simulink model "Energy_Cost"  (Simulink 8.8)
settings: Solver=ode23t  StartTime=0.0  StopTime=24  RelTol=1e-3  EnableMultiTasking=on
model workspace: external: MAT-File (data not in the file)
libraries: simulink x4
(part 1 of 5)
settings Model: Creator=jm3gonza  LastModifiedBy=Lenio
settings DataIOCC: LimitDataPoints=off  SaveOutput=off
settings OptimizationCC: ExpressionDepthLimit=2147483647
settings DebuggingCC: AlgebraicLoopMsg=none  UnconnectedInputMsg=none  UnconnectedOutputMsg=none  UnconnectedLineMsg=none

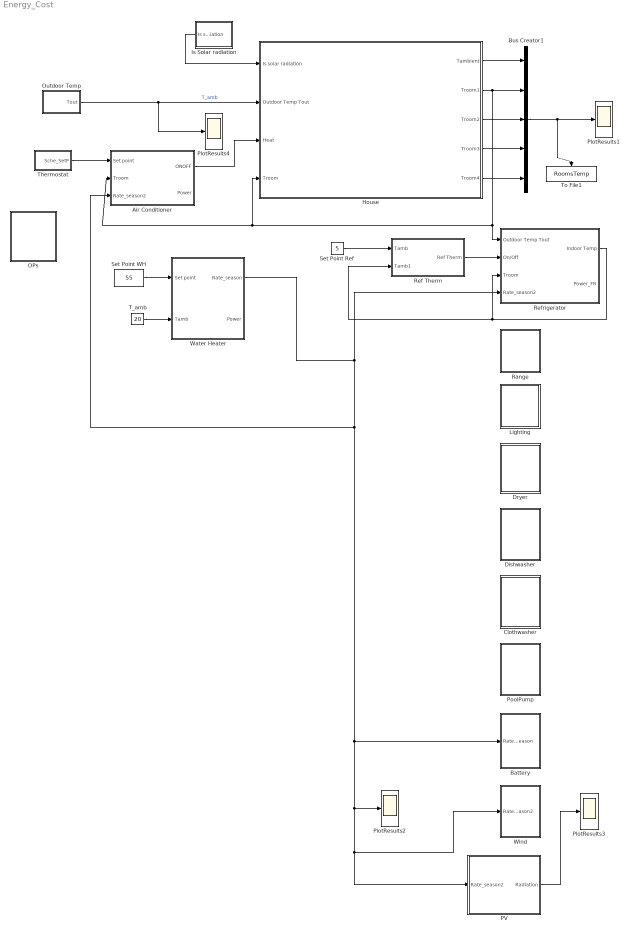
== system Energy_Cost ==
  Air Conditioner : Subsystem
  Battery : Subsystem
  Bus Creator1 : BusCreator  Inputs=5
  Clothwasher : Subsystem
  Dishwasher : Subsystem
  Dryer : Subsystem
  House : Subsystem
  Is Solar radiation : Subsystem
  Lighting : Subsystem
  OPs : Subsystem
  Outdoor Temp : Subsystem
  PV : Subsystem
  PlotResults{1..4} (4 alike) : Scope
  PoolPump : Subsystem
  Range : Subsystem
  Ref Therm : Subsystem
  Refrigerator : Subsystem
  Set Point Ref : Constant  Value=5
  Set Point WH : Constant  Value=55
  T_amb : Constant  Value=20
  Thermostat : Subsystem
  To File1 : ToFile  Filename=RoomsTemp  MatrixName=RoomsTemp
  Water Heater : Subsystem
  Wind : Subsystem
  wires:
  Set Point WH/1 -> Water Heater/1(Set point)
  T_amb/1 -> Water Heater/2(Tamb)
  Outdoor Temp/1(Tout) -> PlotResults4/1, House/2(Outdoor Temp Tout)  "T_amb"
  House/5(Troom4) -> Bus Creator1/5
  House/1(Tambient) -> Bus Creator1/1
  House/2(Troom1) -> Bus Creator1/2, Refrigerator/1(Outdoor Temp Tout), House/4(Troom), Air Conditioner/2(Troom)
  House/3(Troom2) -> Bus Creator1/3
  House/4(Troom3) -> Bus Creator1/4
  Bus Creator1/1 -> To File1/1, PlotResults1/1
  Air Conditioner/1(ONOFF) -> House/3(Heat)
  Is Solar radiation/1(Is solar radiation) -> House/1(Is solar radiation)
  Thermostat/1(Sche_SetP) -> Air Conditioner/1(Set point)
  Set Point Ref/1 -> Ref Therm/1(Tamb)
  Ref Therm/1(Ref Therm) -> Refrigerator/2(On/Off)
  Refrigerator/1(Indoor Temp) -> Refrigerator/3(Troom), Ref Therm/2(Tamb1)
  Water Heater/1(Rate_season) -> Refrigerator/4(Rate_season2), Air Conditioner/3(Rate_season2), Wind/1(Rate_season2), PV/1(Rate_season2), PlotResults2/1, Battery/1(Rate_season)
  PV/1(Radiation) -> PlotResults3/1

== system Energy_Cost/Air Conditioner ==
  Set point : Inport
  Troom : Inport  Port=2
  Rate_season2 : Inport  Port=3
  AA or Heat : Constant
  AA_OnOff : Constant
  Cost_AA : Subsystem
  PlotResults4 : Scope
  Q_AC : Constant  Value=-50644783.1184
  Relay : Relay  OnSwitchValue=0.5  OffSwitchValue=-0.5
  Sum : Sum  Inputs=|+-  SampleTime=0  SaturateOnIntegerOverflow=on  InputSameDT=on  OutDataTypeStr=Inherit: Same as first input
  a : Product  Inputs=3  RndMeth=Zero
  ONOFF : Outport  InitialOutput=0
  Power : Outport  Port=2  InitialOutput=0
  wires:
  Set point/1 -> Sum/1
  Troom/1 -> Sum/2
  Sum/1 -> Relay/1
  Relay/1 -> a/1, PlotResults4/1
  a/1 -> ONOFF/1, Cost_AA/1(Powe_cons)
  Q_AC/1 -> a/2
  AA_OnOff/1 -> a/3
  Rate_season2/1 -> Cost_AA/2(Rate_season2)
  Cost_AA/1(Power) -> Power/1

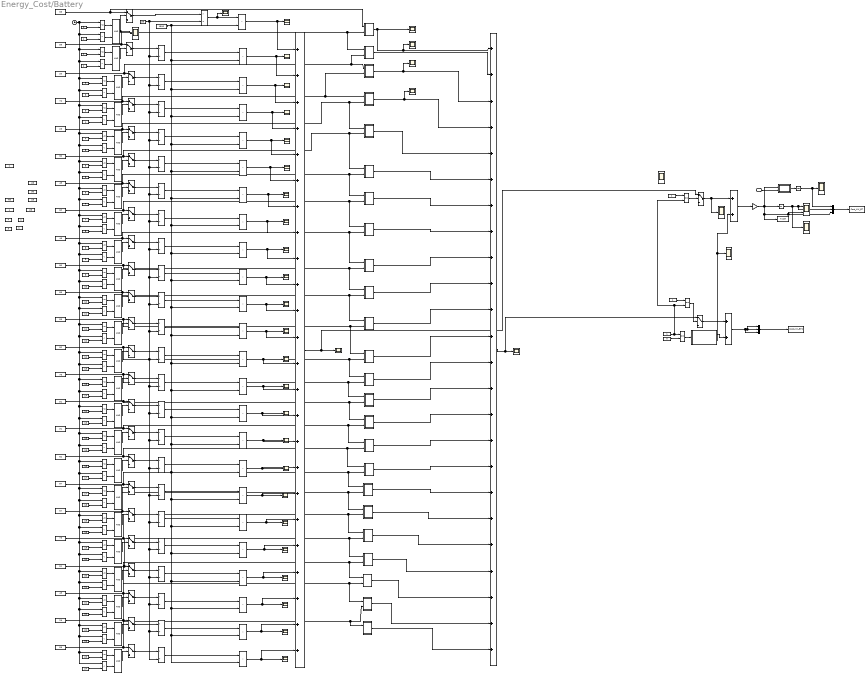
== system Energy_Cost/Battery ==
  Rate_season : Inport
  Add1 : Sum  Inputs=++++++++++++++++++++++++
  Add2 : Sum  Inputs=++++++++++++++++++++++++
  Add8 : Sum
  Add9 : Sum
  BT_OnOff : Constant
  Battery_type : Constant
  Bus Creator1 : BusCreator  Inputs=3
  Bus Creator4 : BusCreator  Inputs=3
  Clock1 : Clock
  Default : Constant  Value=0
  Divide{2..25} (24 alike) : Product  Inputs=*/
  Dot Product{1,3..25} (24 alike) : DotProduct  InputSameDT=on  OutDataTypeStr=Inherit: Inherit via internal rule
  Enabled Subsystem1 : Subsystem  TreatAsAtomicUnit=on
  Gain : Gain  Gain=.001
  Integrator : Integrator
  Integrator3 : Integrator
  Load Value : Constant  Value=-60
  LoadsDay : Constant
  Logical Operator{1..18,20..25} (24 alike) : Logic  AllPortsSameDT=off  OutDataTypeStr=boolean
  MinOfLoad : Constant  Value=30
  PlotResults{1..4,6,8} (6 alike) : Scope
  PlotResults5 : Scope  NumInputPorts=2
  Power1 : Constant  Value=35
  Power10 : Constant  Value=80
  Power11 : Constant  Value=85
  Power12 : Constant  Value=55
  Power13 : Constant  Value=92
  Power14 : Constant  Value=76
  Power15 : Constant  Value=51
  Power16 : Constant  Value=31
  Power17 : Constant  Value=62
  Power18 : Constant  Value=87
  Power19 : Constant  Value=97
  Power2 : Constant  Value=55
  Power20 : Constant  Value=75
  Power21 : Constant  Value=61
  Power22 : Constant  Value=43
  Power23 : Constant  Value=29
  Power24 : Constant  Value=59
  Power25 : Constant  Value=1500
  Power3 : Constant  Value=20
  Power4 : Constant  Value=70
  Power5 : Constant  Value=25
  Power6 : Constant  Value=30
  Power7 : Constant  Value=45
  Power8 : Constant  Value=60
  Power9 : Constant  Value=45
  Rates : Subsystem
  Relational Operator1 : RelationalOperator  Operator===  RndMeth=Nearest  InputSameDT=on
  Relational Operator{6..7,10..11,14..15,18..19,22..23,27..28,31..32,35..36,39..40,43..44,47..48,51..52} (24 alike) : RelationalOperator  RndMeth=Nearest  InputSameDT=on
  Relational Operator103 : RelationalOperator  Operator===  RndMeth=Nearest  InputSameDT=on
  Relational Operator{8..9,12..13,16..17,20..21,25..26,29..30,33..34,37..38,41..42,45..46,49..50,53..54} (24 alike) : RelationalOperator  Operator=<  RndMeth=Nearest  InputSameDT=on
  Relational Operator55 : RelationalOperator  Operator===  RndMeth=Nearest  InputSameDT=on
  Subsystem : Subsystem
  Subsystem1 : Subsystem
  Subsystem10 : Subsystem
  Subsystem11 : Subsystem
  Subsystem12 : Subsystem
  Subsystem13 : Subsystem
  Subsystem14 : Subsystem
  Subsystem15 : Subsystem
  Subsystem16 : Subsystem
  Subsystem17 : Subsystem
  Subsystem18 : Subsystem
  Subsystem19 : Subsystem
  Subsystem2 : Subsystem
  Subsystem20 : Subsystem
  Subsystem21 : Subsystem
  Subsystem22 : Subsystem
  Subsystem23 : Subsystem
  Subsystem3 : Subsystem
  Subsystem4 : Subsystem
  Subsystem5 : Subsystem
  Subsystem6 : Subsystem
  Subsystem7 : Subsystem
  Subsystem8 : Subsystem
  Subsystem9 : Subsystem
  Switch{1,7..29,31..32} (26 alike) : Switch  Criteria=u2 > Threshold
  To File1 : ToFile  Filename=TinBT  MatrixName=TinBT
  To File3 : ToFile  Filename=Cost_KW_BT2  MatrixName=Cost_KW_BT2
  To File5 : ToFile  Filename=Cost_KW_BT  MatrixName=Cost_KW_BT
  Type1 : Constant
  Type10 : Constant  Value=2
  Type11 : Constant  Value=3
  Type12 : Constant  Value=4
  Type13 : Constant  Value=4
  Type14 : Constant  Value=5
  Type15 : Constant  Value=6
  Type16 : Constant  Value=5
  Type17 : Constant  Value=6
  Type18 : Constant  Value=7
  Type19 : Constant  Value=8
  Type2 : Constant  Value=2
  Type20 : Constant  Value=8
  Type21 : Constant  Value=9
  Type22 : Constant  Value=10
  Type23 : Constant  Value=9
  Type24 : Constant  Value=7
  Type25 : Constant  Value=10
  Type26 : Constant  Value=11
  Type27 : Constant  Value=12
  Type28 : Constant  Value=12
  Type29 : Constant  Value=13
  Type3 : Constant  Value=3
  Type30 : Constant  Value=14
  Type31 : Constant  Value=13
  Type32 : Constant  Value=14
  Type33 : Constant  Value=15
  Type34 : Constant  Value=16
  Type35 : Constant  Value=16
  Type36 : Constant  Value=17
  Type37 : Constant  Value=18
  Type38 : Constant  Value=17
  Type39 : Constant  Value=15
  Type4 : Constant  Value=4
  Type40 : Constant  Value=11
  Type41 : Constant  Value=18
  Type42 : Constant  Value=19
  Type43 : Constant  Value=20
  Type44 : Constant  Value=20
  Type45 : Constant  Value=21
  Type46 : Constant  Value=22
  Type47 : Constant  Value=21
  Type48 : Constant  Value=22
  Type49 : Constant  Value=23
  Type5 : Constant
  Type50 : Constant  Value=24
  Type52 : Constant  Value=35
  Type55 : Constant  Value=23
  Type56 : Constant  Value=19
  Type6 : Constant  Value=0
  Type7 : Constant
  Type8 : Constant  Value=2
  Type9 : Constant  Value=3
  WhenUsed1 : Constant  Value=25
  WhenUsed2 : Constant  Value=25
  WhenUsed3 : Constant  Value=25
  radiation : Constant
  radiation1 : Constant
  scope{1..26} (26 alike) : Scope
  soc{,1..4} (5 alike) : Scope
  wires:
  Integrator/1 -> Bus Creator4/1, PlotResults3/1
  Rates/1(Rate) -> Integrator/1
  Integrator3/1 -> PlotResults6/1, Bus Creator4/2, PlotResults5/1  "kw-hr"
  Bus Creator4/1 -> To File5/1
  Rate_season/1 -> Rates/2(Rate_season)
  Bus Creator1/1 -> To File3/1
  Default/1 -> Relational Operator103/2
  Relational Operator103/1 -> Enabled Subsystem1/1(active pulse1)
  Relational Operator55/1 -> Switch29/2
  radiation/1 -> Relational Operator55/1
  Switch29/1 -> Add8/1
  Gain/1 -> PlotResults5/2, Bus Creator4/3, To File1/1, Integrator3/1, Rates/1(Powe_cons)
  Switch1/1 -> Add9/1, PlotResults8/1
  radiation1/1 -> Relational Operator1/1
  Relational Operator1/1 -> Switch1/2
  Add8/1 -> Bus Creator1/2, Bus Creator1/1, Bus Creator1/3
  Add9/1 -> Gain/1
  Type36/1 -> Relational Operator41/2
  Relational Operator41/1 -> Logical Operator18/2
  Type38/1 -> Relational Operator39/2
  Type37/1 -> Relational Operator42/2
  Relational Operator42/1 -> Logical Operator11/2
  Relational Operator39/1 -> Logical Operator11/1
  Logical Operator11/1 -> Switch21/2
  Type41/1 -> Relational Operator44/2
  Type42/1 -> Relational Operator45/2
  Relational Operator45/1 -> Logical Operator20/2
  Relational Operator44/1 -> Logical Operator20/1
  Logical Operator20/1 -> Switch32/2
  Type56/1 -> Relational Operator43/2
  Type43/1 -> Relational Operator46/2
  Relational Operator46/1 -> Logical Operator21/2
  Relational Operator43/1 -> Logical Operator21/1
  Logical Operator21/1 -> Switch25/2
  Type44/1 -> Relational Operator48/2
  Type45/1 -> Relational Operator49/2
  Relational Operator49/1 -> Logical Operator22/2
  Relational Operator48/1 -> Logical Operator22/1
  Logical Operator22/1 -> Switch27/2
  Type47/1 -> Relational Operator47/2
  Type46/1 -> Relational Operator50/2
  Relational Operator50/1 -> Logical Operator23/2
  Relational Operator47/1 -> Logical Operator23/1
  Logical Operator23/1 -> Switch26/2
  Type48/1 -> Relational Operator52/2
  Type49/1 -> Relational Operator53/2
  Relational Operator53/1 -> Logical Operator24/2
  Relational Operator52/1 -> Logical Operator24/1
  Logical Operator24/1 -> Switch31/2
  Type55/1 -> Relational Operator51/2
  Type50/1 -> Relational Operator54/2
  Relational Operator54/1 -> Logical Operator25/2
  Relational Operator51/1 -> Logical Operator25/1
  Logical Operator25/1 -> Switch28/2
  Power18/1 -> Switch21/1, Subsystem16/2(In2), Subsystem17/1(In1)
  Power19/1 -> Switch32/1, Subsystem17/2(In2), Subsystem18/1(In1)
  Power20/1 -> Switch25/1, Subsystem18/2(In2), Subsystem19/1(In1)
  Power21/1 -> Switch27/1, Subsystem19/2(In2), Subsystem20/1(In1)
  Power22/1 -> Switch26/1, Subsystem20/2(In2), Subsystem21/1(In1)
  Power23/1 -> Switch31/1, Subsystem21/2(In2), Subsystem22/1(In1)
  Power24/1 -> Switch28/1, Subsystem22/2(In2), Subsystem23/1(In1)
  Power1/1 -> Switch7/1, Subsystem/1(In1)
  Switch7/1 -> Divide2/1
  Clock1/1 -> Relational Operator7/1, Relational Operator8/1, Relational Operator6/1, Relational Operator9/1, Relational Operator11/1, Relational Operator19/1, Relational Operator20/1, Relational Operator18/1, Relational Operator21/1, Relational Operator23/1, Relational Operator25/1, Relational Operator22/1, Relational Operator26/1, Relational Operator28/1, Relational Operator29/1, Relational Operator27/1, Relational Operator32/1, Relational Operator31/1, Relational Operator34/1, Relational Operator36/1, Relational Operator37/1, Relational Operator35/1, Relational Operator38/1, Relational Operator40/1, Relational Operator41/1, Relational Operator39/1, Relational Operator42/1, Relational Operator45/1, Relational Operator43/1, Relational Operator47/1, Relational Operator54/1, Relational Operator51/1, Relational Operator53/1, Relational Operator52/1, Relational Operator50/1, Relational Operator49/1, Relational Operator48/1, Relational Operator46/1, Relational Operator44/1, Relational Operator33/1, Relational Operator30/1, Relational Operator17/1, Relational Operator14/1, Relational Operator16/1, Relational Operator15/1, Relational Operator13/1, Relational Operator10/1, Relational Operator12/1
  Type6/1 -> Relational Operator7/2
  Relational Operator7/1 -> Logical Operator1/1
  Power2/1 -> Switch8/1, Subsystem/2(In2), Subsystem1/1(In1)
  Type5/1 -> Relational Operator6/2
  Relational Operator6/1 -> Logical Operator2/1
  Type10/1 -> Relational Operator11/2
  Relational Operator11/1 -> Logical Operator3/1
  Type9/1 -> Relational Operator10/2
  Type12/1 -> Relational Operator13/2
  Relational Operator13/1 -> Logical Operator4/2
  Relational Operator10/1 -> Logical Operator4/1
  Logical Operator4/1 -> Switch10/2
  Type13/1 -> Relational Operator15/2
  Type14/1 -> Relational Operator16/2
  Relational Operator16/1 -> Logical Operator5/2
  Relational Operator15/1 -> Logical Operator5/1
  Logical Operator5/1 -> Switch12/2
  Type16/1 -> Relational Operator14/2
  Type15/1 -> Relational Operator17/2
  Relational Operator17/1 -> Logical Operator6/2
  Relational Operator14/1 -> Logical Operator6/1
  Logical Operator6/1 -> Switch11/2
  Type17/1 -> Relational Operator19/2
  Type18/1 -> Relational Operator20/2
  Relational Operator20/1 -> Logical Operator7/2
  Relational Operator19/1 -> Logical Operator7/1
  Logical Operator7/1 -> Switch16/2
  Type24/1 -> Relational Operator18/2
  Type19/1 -> Relational Operator21/2
  Relational Operator21/1 -> Logical Operator8/2
  Relational Operator18/1 -> Logical Operator8/1
  Logical Operator8/1 -> Switch13/2
  Type20/1 -> Relational Operator23/2
  Type21/1 -> Relational Operator25/2
  Relational Operator25/1 -> Logical Operator9/2
  Relational Operator23/1 -> Logical Operator9/1
  Logical Operator9/1 -> Switch15/2
  Type23/1 -> Relational Operator22/2
  Type22/1 -> Relational Operator26/2
  Relational Operator26/1 -> Logical Operator10/2
  Relational Operator22/1 -> Logical Operator10/1
  Logical Operator10/1 -> Switch14/2
  Type25/1 -> Relational Operator28/2
  Type26/1 -> Relational Operator29/2
  Relational Operator29/1 -> Logical Operator12/2
  Relational Operator28/1 -> Logical Operator12/1
  Logical Operator12/1 -> Switch24/2
  Type40/1 -> Relational Operator27/2
  Type27/1 -> Relational Operator30/2
  Relational Operator30/1 -> Logical Operator13/2
  Relational Operator27/1 -> Logical Operator13/1
  Logical Operator13/1 -> Switch17/2
  Type28/1 -> Relational Operator32/2
  Type29/1 -> Relational Operator33/2
  Relational Operator33/1 -> Logical Operator14/2
  Relational Operator32/1 -> Logical Operator14/1
  Logical Operator14/1 -> Switch19/2
  Type31/1 -> Relational Operator31/2
  Type30/1 -> Relational Operator34/2
  Relational Operator34/1 -> Logical Operator15/2
  Relational Operator31/1 -> Logical Operator15/1
  Logical Operator15/1 -> Switch18/2
  Type32/1 -> Relational Operator36/2
  Type33/1 -> Relational Operator37/2
  Relational Operator37/1 -> Logical Operator16/2
  Relational Operator36/1 -> Logical Operator16/1
  Logical Operator16/1 -> Switch23/2
  Type39/1 -> Relational Operator35/2
  Type34/1 -> Relational Operator38/2
  Relational Operator38/1 -> Logical Operator17/2
  Relational Operator35/1 -> Logical Operator17/1
  Logical Operator17/1 -> Switch20/2
  Type35/1 -> Relational Operator40/2
  Relational Operator40/1 -> Logical Operator18/1
  Logical Operator18/1 -> Switch22/2
  Power3/1 -> Switch9/1, Subsystem1/2(In2), Subsystem2/1(In1)
  Power4/1 -> Switch10/1, Subsystem2/2(In2), Subsystem3/1(In1)
  Power5/1 -> Switch12/1, Subsystem3/2(In2), Subsystem4/1(In1)
  Power6/1 -> Switch11/1, Subsystem4/2(In2), Subsystem5/1(In1)
  Power7/1 -> Switch16/1, Subsystem5/2(In2), Subsystem6/1(In1)
  Power8/1 -> Switch13/1, Subsystem6/2(In2), Subsystem7/1(In1)
  Power9/1 -> Switch15/1, Subsystem7/2(In2), Subsystem8/1(In1)
  Power10/1 -> Switch14/1, Subsystem8/2(In2), Subsystem9/1(In1)
  Power11/1 -> Switch24/1, Subsystem9/2(In2), Subsystem10/1(In1)
  Power12/1 -> Switch17/1, Subsystem10/2(In2), Subsystem11/1(In1)
  Power13/1 -> Switch19/1, Subsystem11/2(In2), Subsystem12/1(In1)
  Power14/1 -> Switch18/1, Subsystem12/2(In2), Subsystem13/1(In1)
  Power15/1 -> Switch23/1, Subsystem13/2(In2), Subsystem14/1(In1)
  Power16/1 -> Switch20/1, Subsystem14/2(In2), Subsystem15/1(In1)
  Power17/1 -> Switch22/1, Subsystem15/2(In2), Subsystem16/1(In1)
  Type52/1 -> Divide2/2, Divide3/2, Divide4/2, Divide5/2, Divide9/2, Divide10/2, Divide12/2, Divide13/2, Divide18/2, Divide19/2, Divide20/2, Divide21/2, Divide22/2, Divide23/2, Divide25/2, Divide24/2, Divide17/2, Divide16/2, Divide15/2, Divide14/2, Divide11/2, Divide8/2, Divide7/2, Divide6/2
  Divide2/1 -> Dot Product1/1, scope2/1
  Power25/1 -> Dot Product1/2, Dot Product3/2, Dot Product4/2, Dot Product6/2, Dot Product7/2, Dot Product12/2, Dot Product13/2, Dot Product14/2, Dot Product18/2, Dot Product19/2, Dot Product20/2, Dot Product21/2, Dot Product22/2, Dot Product23/2, Dot Product25/2, Dot Product24/2, Dot Product17/2, Dot Product16/2, Dot Product15/2, Dot Product11/2, Dot Product10/2, Dot Product9/2, Dot Product8/2, Dot Product5/2
  Dot Product1/1 -> scope1/1, Add2/1
  Switch8/1 -> Divide3/1
  Divide3/1 -> Dot Product3/1
  Dot Product3/1 -> scope3/1, Add2/2
  Divide4/1 -> Dot Product4/1
  Dot Product4/1 -> scope4/1, Add2/3
  Divide5/1 -> Dot Product5/1
  Dot Product5/1 -> scope5/1, Add2/4
  Divide6/1 -> Dot Product6/1
  Dot Product6/1 -> scope6/1, Add2/5
  Divide7/1 -> Dot Product7/1
  Dot Product7/1 -> scope7/1, Add2/6
  Divide8/1 -> Dot Product8/1
  Dot Product8/1 -> scope8/1, Add2/7
  Divide9/1 -> Dot Product9/1
  Dot Product9/1 -> scope9/1, Add2/8
  Divide10/1 -> Dot Product10/1
  Dot Product10/1 -> scope10/1, Add2/9
  Divide11/1 -> Dot Product11/1
  Dot Product11/1 -> scope11/1, Add2/10
  Divide12/1 -> Dot Product12/1
  Dot Product12/1 -> scope12/1, Add2/11
  Divide13/1 -> Dot Product13/1
  Dot Product13/1 -> scope13/1, Add2/12
  Divide14/1 -> Dot Product14/1
  Dot Product14/1 -> scope14/1, Add2/13
  Divide15/1 -> Dot Product15/1
  Dot Product15/1 -> scope15/1, Add2/14
  Divide16/1 -> Dot Product16/1
  Dot Product16/1 -> scope16/1, Add2/15
  Divide17/1 -> Dot Product17/1
  Dot Product17/1 -> scope17/1, Add2/16
  Divide18/1 -> Dot Product18/1
  Dot Product18/1 -> scope18/1, Add2/17
  Divide19/1 -> Dot Product19/1
  Dot Product19/1 -> scope19/1, Add2/18
  Divide20/1 -> Dot Product20/1
  Dot Product20/1 -> scope20/1, Add2/19
  Divide21/1 -> Dot Product21/1
  Dot Product21/1 -> scope21/1, Add2/20
  Divide22/1 -> Dot Product22/1
  Dot Product22/1 -> scope22/1, Add2/21
  Divide23/1 -> Dot Product23/1
  Dot Product23/1 -> scope23/1, Add2/22
  Divide24/1 -> Dot Product24/1
  Dot Product24/1 -> scope24/1, Add2/23
  Divide25/1 -> Dot Product25/1
  Dot Product25/1 -> scope25/1, Add2/24
  Switch28/1 -> Divide25/1
  Switch31/1 -> Divide24/1
  Switch26/1 -> Divide23/1
  Switch27/1 -> Divide22/1
  Switch25/1 -> Divide21/1
  Switch32/1 -> Divide20/1
  Switch21/1 -> Divide19/1
  Switch22/1 -> Divide18/1
  Switch20/1 -> Divide17/1
  Switch23/1 -> Divide16/1
  Switch18/1 -> Divide15/1
  Switch19/1 -> Divide14/1
  Switch17/1 -> Divide13/1
  Switch24/1 -> Divide12/1
  Switch14/1 -> Divide11/1
  Switch15/1 -> Divide10/1
  Switch13/1 -> Divide9/1
  Switch16/1 -> Divide8/1
  Switch11/1 -> Divide7/1
  Switch12/1 -> Divide6/1
  Switch10/1 -> Divide5/1
  Switch9/1 -> Divide4/1
  Add2/1 -> scope26/1, Switch1/1
  Logical Operator3/1 -> Switch9/2
  Relational Operator12/1 -> Logical Operator3/2
  Type11/1 -> Relational Operator12/2
  Logical Operator2/1 -> Switch8/2
  Type8/1 -> Relational Operator9/2
  Relational Operator9/1 -> Logical Operator2/2
  Logical Operator1/1 -> Switch7/2, PlotResults4/1
  Type7/1 -> Relational Operator8/2
  Relational Operator8/1 -> Logical Operator1/2
  Subsystem/1(Out1) -> soc1/1, Add1/1, soc2/1
  Subsystem1/1(Out1) -> Add1/2
  Subsystem2/1(Out1) -> soc3/1, Add1/3
  Subsystem3/1(Out1) -> Add1/4, soc4/1
  Add1/1 -> soc/1, Switch29/1
  Subsystem4/1(Out1) -> Add1/5
  Subsystem5/1(Out1) -> Add1/6
  Subsystem6/1(Out1) -> Add1/7
  Subsystem7/1(Out1) -> Add1/8
  Subsystem8/1(Out1) -> Add1/9
  Subsystem9/1(Out1) -> Add1/10
  Subsystem10/1(Out1) -> Add1/11
  Subsystem11/1(Out1) -> Add1/12
  Subsystem12/1(Out1) -> Add1/13
  Subsystem13/1(Out1) -> Add1/14
  Subsystem14/1(Out1) -> Add1/15
  Subsystem15/1(Out1) -> Add1/16
  Subsystem16/1(Out1) -> Add1/17
  Subsystem17/1(Out1) -> Add1/18
  Subsystem18/1(Out1) -> Add1/19
  Subsystem19/1(Out1) -> Add1/20
  Subsystem20/1(Out1) -> Add1/21
  Subsystem21/1(Out1) -> Add1/22
  Subsystem22/1(Out1) -> Add1/23
  Subsystem23/1(Out1) -> Add1/24
  Enabled Subsystem1/1(SOC) -> Add8/2
  Enabled Subsystem1/2(Power) -> Add9/2, PlotResults2/1
  BT_OnOff/1 -> Relational Operator103/1, Relational Operator55/2, Relational Operator1/2

== system Energy_Cost/Clothwasher ==
  AnnualPower : Constant  Value=154
  Bus Creator : BusCreator  Inputs=10
  DW_OnOff : Constant
  LoadsDay : Constant  Value=3
  MinOfLoad : Constant  Value=60
  Terminator : Terminator
  TypeDW : Constant
  WH conected : Constant  Value=0
  WaterTemp : Constant
  WhenUsed1 : Constant  Value=8
  WhenUsed2 : Constant  Value=13
  WhenUsed3 : Constant  Value=18
  wires:
  AnnualPower/1 -> Bus Creator/2
  LoadsDay/1 -> Bus Creator/3
  MinOfLoad/1 -> Bus Creator/4
  WhenUsed1/1 -> Bus Creator/5
  WhenUsed2/1 -> Bus Creator/6
  WhenUsed3/1 -> Bus Creator/7
  DW_OnOff/1 -> Bus Creator/1
  Bus Creator/1 -> Terminator/1
  TypeDW/1 -> Bus Creator/8
  WH conected/1 -> Bus Creator/9
  WaterTemp/1 -> Bus Creator/10

== system Energy_Cost/Dishwasher ==
  AnnualPower : Constant  Value=250
  Bus Creator : BusCreator  Inputs=9
  DW_OnOff : Constant
  LoadsDay : Constant  Value=3
  MinOfLoad : Constant  Value=120
  Terminator : Terminator
  TypeDW : Constant
  WH conected : Constant  Value=0
  WhenUsed1 : Constant  Value=10
  WhenUsed2 : Constant  Value=15
  WhenUsed3 : Constant  Value=21.5
  wires:
  AnnualPower/1 -> Bus Creator/2
  LoadsDay/1 -> Bus Creator/3
  MinOfLoad/1 -> Bus Creator/4
  WhenUsed1/1 -> Bus Creator/5
  WhenUsed2/1 -> Bus Creator/6
  WhenUsed3/1 -> Bus Creator/7
  DW_OnOff/1 -> Bus Creator/1
  Bus Creator/1 -> Terminator/1
  TypeDW/1 -> Bus Creator/8
  WH conected/1 -> Bus Creator/9

== system Energy_Cost/Dryer ==
  Bus Creator : BusCreator  Inputs=6
  DY_OnOff : Constant
  LoadsDay : Constant  Value=3
  MinOfLoad : Constant  Value=80
  Terminator : Terminator
  WhenUsed1 : Constant  Value=10
  WhenUsed2 : Constant  Value=15
  WhenUsed3 : Constant  Value=20
  wires:
  DY_OnOff/1 -> Bus Creator/1
  Bus Creator/1 -> Terminator/1
  WhenUsed3/1 -> Bus Creator/6
  WhenUsed2/1 -> Bus Creator/5
  WhenUsed1/1 -> Bus Creator/4
  MinOfLoad/1 -> Bus Creator/3
  LoadsDay/1 -> Bus Creator/2

== system Energy_Cost/House ==
  Is solar radiation : Inport
  Outdoor Temp Tout : Inport  Port=2
  Heat : Inport  Port=3
  Troom : Inport  Port=4
  Room_1 : Subsystem
  Room_2 : Subsystem
  Room_3 : Subsystem
  Room_4 : Subsystem
  Tambient : Outport  InitialOutput=0
  Troom1 : Outport  Port=2  InitialOutput=0
  Troom2 : Outport  Port=3  InitialOutput=0
  Troom3 : Outport  Port=4  InitialOutput=0
  Troom4 : Outport  Port=5  InitialOutput=0
  wires:
  Is solar radiation/1 -> Room_1/1(Is solar radiation), Room_2/1(Is solar radiation), Room_3/1(Is solar radiation), Room_4/1(Is solar radiation)
  Outdoor Temp Tout/1 -> Room_1/2(Outdoor Temp Tout), Room_2/2(Outdoor Temp Tout), Room_3/2(Outdoor Temp Tout), Room_4/2(Outdoor Temp Tout), Tambient/1
  Heat/1 -> Room_1/3(Q_Heat), Room_2/3(Q_Heat), Room_3/3(Q_Heat), Room_4/3(Q_Heat)  "Q_Heat"
  Troom/1 -> Room_1/4(Troom), Room_2/4(Troom), Room_3/4(Troom), Room_4/4(Troom)
  Room_1/1(Room Temp Troom) -> Troom1/1
  Room_2/1(Room Temp Troom) -> Troom2/1
  Room_3/1(Room Temp Troom) -> Troom3/1
  Room_4/1(Room Temp Troom) -> Troom4/1

== system Energy_Cost/Is Solar radiation ==
  Avg Outdoor Temp : Constant
  Outdoor Temp : simulink/Sources/Repeating Sequence Interpolated  OutValues=|  TimeValues=|  LookUpMeth=Interpolation-Use End Values  tsamp=-1  OutMin=[]  OutMax=[]  OutDataTypeStr=double  OutputDataTypeScalingMode=double  OutDataType=fixdt(0,8)  OutScaling=2^-10
      OutValues=|
      | [0
      | 0
      | 0
      | 0
      | 0
      | 0
      | 0
      | 0
      | 0
      | 0
      | 0
      | 0
      | 0
      | 0
      | 0
      | 0
      | 0
      | 0
      | 0
      | 0
      | 0
      | 12.85
      | 12.85
      | 12.85
      | 25.699
      | 38.55
      | 51.399
      | 38.55
      | 70.673
      | 70.674
      | 122.073
      | 147.772
      | 102.797
      | 237.697
      | 160.597
      | 186.273
      | 186.268
      | 173.422
      | 404.649
      | 571.658
      | 327.556
      | 411.017
      | 468.811
      | 391.717
      | 314.634
      | 237.577
      | 301.802
      | 417.367
      | 584.316
      | 449.469
      | 719.125
      | 532.917
      | 340.26
      | 199.027
      | 340.266
      | 404.503
      | 288.922
      | 314.601
      | 340.296
      | 301.769
      | 288.938
      | 263.253
      | 288.942
      | 321.049
      | 417.349
      | 327.463
      | 365.947
      | 365.936
      | 269.636
      | 224.709
      | 231.145
      | 173.362
      | 154.103
      | 147.682
      | 128.422
      | 102.737
      | 83.473
      | 70.634
      | 25.685
      | 25.686
      | 0
      | 0
      | 0
      | 0
      | 0
      | 0
      | 0
      | 0
      | 0
      | 0
      | 0
      | 0
      | 0
      | 0
      | 0
      | 0
      | ].'
      TimeValues=|
      | [         0
      |     0.1500
      |     0.3000
      |     0.4500
      |     1.0000
      |     1.1500
      |     1.3000
      |     1.4500
      |     2.0000
      |     2.1500
      |     2.3000
      |     2.4500
      |     3.0000
      |     3.1500
      |     3.3000
      |     3.4500
      |     4.0000
      |     4.1500
      |     4.3000
      |     4.4500
      |     5.0000
      |     5.1500
      |     5.3000
      |     5.4500
      |     6.0000
      |     6.1500
      |     6.3000
      |     6.4500
      |     7.0000
      |     7.1500
      |     7.3000
      |     7.4500
      |     8.0000
      |     8.1500
      |     8.3000
      |     8.4500
      |     9.0000
      |     9.1500
      |     9.3000
      |     9.4500
      |    10.0000
      |    10.1500
      |    10.3000
      |    10.4500
      |    11.0000
      |    11.1500
      |    11.3000
      |    11.4500
      |    12.0000
      |    12.1500
      |    12.3000
      |    12.4500
      |    13.0000
      |    13.1500
      |    13.3000
      |    13.4500
      |    14.0000
      |    14.1500
      |    14.3000
      |    14.4500
      |    15.0000
      |    15.1500
      |    15.3000
      |    15.4500
      |    16.0000
      |    16.1500
      |    16.3000
      |    16.4500
      |    17.0000
      |    17.1500
      |    17.3000
      |    17.4500
      |    18.0000
      |    18.1500
      |    18.3000
      |    18.4500
      |    19.0000
      |    19.1500
      |    19.3000
      |    19.4500
      |    20.0000
      |    20.1500
      |    20.3000
      |    20.4500
      |    21.0000
      |    21.1500
      |    21.3000
      |    21.4500
      |    22.0000
      |    22.1500
      |    22.3000
      |    22.4500
      |    23.0000
      |    23.1500
      |    23.3000
      |    23.4500].'
  Sum1 : Sum  Inputs=|++  SaturateOnIntegerOverflow=on  InputSameDT=on  OutDataTypeStr=Inherit: Same as first input
  Is solar radiation : Outport  InitialOutput=0
  wires:
  Avg Outdoor Temp/1 -> Sum1/1
  Outdoor Temp/1 -> Sum1/2
  Sum1/1 -> Is solar radiation/1

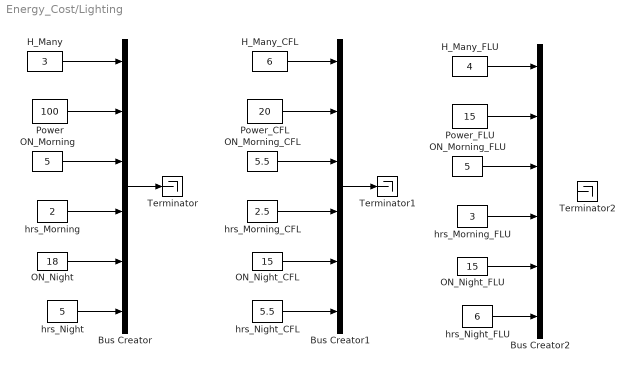
== system Energy_Cost/Lighting ==
  Bus Creator : BusCreator  Inputs=6
  Bus Creator1 : BusCreator  Inputs=6
  Bus Creator2 : BusCreator  Inputs=6
  H_Many : Constant  Value=3
  H_Many_CFL : Constant  Value=6
  H_Many_FLU : Constant  Value=4
  ON_Morning : Constant  Value=5
  ON_Morning_CFL : Constant  Value=5.5
  ON_Morning_FLU : Constant  Value=5
  ON_Night : Constant  Value=18
  ON_Night_CFL : Constant  Value=15
  ON_Night_FLU : Constant  Value=15
  Power : Constant  Value=100
  Power_CFL : Constant  Value=20
  Power_FLU : Constant  Value=15
  Terminator : Terminator
  Terminator1 : Terminator
  Terminator2 : Terminator
  hrs_Morning : Constant  Value=2
  hrs_Morning_CFL : Constant  Value=2.5
  hrs_Morning_FLU : Constant  Value=3
  hrs_Night : Constant  Value=5
  hrs_Night_CFL : Constant  Value=5.5
  hrs_Night_FLU : Constant  Value=6
  wires:
  Bus Creator/1 -> Terminator/1
  H_Many/1 -> Bus Creator/1
  Power/1 -> Bus Creator/2
  ON_Morning/1 -> Bus Creator/3
  hrs_Morning/1 -> Bus Creator/4
  ON_Night/1 -> Bus Creator/5
  hrs_Night/1 -> Bus Creator/6
  H_Many_CFL/1 -> Bus Creator1/1
  Power_CFL/1 -> Bus Creator1/2
  ON_Morning_CFL/1 -> Bus Creator1/3
  hrs_Morning_CFL/1 -> Bus Creator1/4
  ON_Night_CFL/1 -> Bus Creator1/5
  hrs_Night_CFL/1 -> Bus Creator1/6
  Bus Creator1/1 -> Terminator1/1
  H_Many_FLU/1 -> Bus Creator2/1
  Power_FLU/1 -> Bus Creator2/2
  ON_Morning_FLU/1 -> Bus Creator2/3
  hrs_Morning_FLU/1 -> Bus Creator2/4
  ON_Night_FLU/1 -> Bus Creator2/5
  hrs_Night_FLU/1 -> Bus Creator2/6

== system Energy_Cost/OPs ==
  Bus Creator : BusCreator  Inputs=6
  Dishwasher_OP : Constant  Value=0
  Dryer_OP : Constant  Value=0
  EveryOP : Constant
  Lighting_OP : Constant  Value=0
  Stove_OP : Constant  Value=0
  Terminator : Terminator
  Washer_OP : Constant  Value=0
  wires:
  Lighting_OP/1 -> Bus Creator/2
  Dryer_OP/1 -> Bus Creator/3
  Dishwasher_OP/1 -> Bus Creator/4
  Washer_OP/1 -> Bus Creator/5
  EveryOP/1 -> Bus Creator/6
  Stove_OP/1 -> Bus Creator/1
  Bus Creator/1 -> Terminator/1

== system Energy_Cost/Outdoor Temp ==
  Heater Switch1 : Product  RndMeth=Zero
  Heater Switch2 : Product  RndMeth=Zero
  Sum2 : Sum  SaturateOnIntegerOverflow=on  InputSameDT=on  OutDataTypeStr=Inherit: Same as first input
  Summer : simulink/Sources/Repeating Sequence Interpolated  OutValues=|  TimeValues=|  LookUpMeth=Interpolation-Use End Values  tsamp=-1  OutMin=[]  OutMax=[]  OutDataTypeStr=double  OutputDataTypeScalingMode=double  OutDataType=fixdt(0,8)  OutScaling=2^-10
      OutValues=|
      | [   23.8160
      |    23.7130
      |    23.4480
      |    23.2590
      |    23.1710
      |    23.1330
      |    22.9330
      |    22.8600
      |    22.7100
      |    22.6330
      |    22.4980
      |    22.3130
      |    22.2390
      |    22.1040
      |    21.9830
      |    21.7030
      |    21.5360
      |    21.4650
      |    21.8150
      |    22.1730
      |    22.3830
      |    22.6540
      |    22.7390
      |    22.9630
      |    23.3760
      |    23.9600
      |    24.3460
      |    24.7420
      |    24.9870
      |    25.3280
      |    25.6220
      |    26.4600
      |    26.8940
      |    27.7100
      |    27.9620
      |    28.1630
      |    28.4950
      |    29.0620
      |    29.0190
      |    29.0170
      |    29.2500
      |    29.6940
      |    29.8860
      |    29.9560
      |    30.0730
      |    30.6760
      |    30.8120
      |    30.9150
      |    31.2920
      |    30.8100
      |    31.3250
      |    31.3570
      |    31.6710
      |    32.3710
      |    31.6010
      |    32.0310
      |    32.1090
      |    32.3180
      |    32.3980
      |    31.7870
      |    31.6290
      |    33.0060
      |    33.0040
      |    32.8570
      |    32.9240
      |    32.6620
      |    33.1210
      |    32.6940
      |    32.3640
      |    32.0100
      |    31.5350
      |    32.0310
      |    31.0020
      |    30.4620
      |    30.0880
      |    29.8870
      |    29.5410
      |    29.3690
      |    29.1040
      |    28.6390
      |    28.1200
      |    26.7970
      |    26.0180
      |    25.6170
      |    26.9460
      |    27.3140
      |    27.1220
      |    26.8170
      |    26.5690
      |    26.4040
      |    26.2680
      |    26.1190
      |    25.7690
      |    25.4730
      |    25.2080
      |    24.9570].'
      TimeValues=|
      | [         0
      |     0.1500
      |     0.3000
      |     0.4500
      |     1.0000
      |     1.1500
      |     1.3000
      |     1.4500
      |     2.0000
      |     2.1500
      |     2.3000
      |     2.4500
      |     3.0000
      |     3.1500
      |     3.3000
      |     3.4500
      |     4.0000
      |     4.1500
      |     4.3000
      |     4.4500
      |     5.0000
      |     5.1500
      |     5.3000
      |     5.4500
      |     6.0000
      |     6.1500
      |     6.3000
      |     6.4500
      |     7.0000
      |     7.1500
      |     7.3000
      |     7.4500
      |     8.0000
      |     8.1500
      |     8.3000
      |     8.4500
      |     9.0000
      |     9.1500
      |     9.3000
      |     9.4500
      |    10.0000
      |    10.1500
      |    10.3000
      |    10.4500
      |    11.0000
      |    11.1500
      |    11.3000
      |    11.4500
      |    12.0000
      |    12.1500
      |    12.3000
      |    12.4500
      |    13.0000
      |    13.1500
      |    13.3000
      |    13.4500
      |    14.0000
      |    14.1500
      |    14.3000
      |    14.4500
      |    15.0000
      |    15.1500
      |    15.3000
      |    15.4500
      |    16.0000
      |    16.1500
      |    16.3000
      |    16.4500
      |    17.0000
      |    17.1500
      |    17.3000
      |    17.4500
      |    18.0000
      |    18.1500
      |    18.3000
      |    18.4500
      |    19.0000
      |    19.1500
      |    19.3000
      |    19.4500
      |    20.0000
      |    20.1500
      |    20.3000
      |    20.4500
      |    21.0000
      |    21.1500
      |    21.3000
      |    21.4500
      |    22.0000
      |    22.1500
      |    22.3000
      |    22.4500
      |    23.0000
      |    23.1500
      |    23.3000
      |    23.4500].'
  Temp_aux : Constant  SampleTime=0
  Temp_aux1 : Constant  Value=0  SampleTime=0
  Winter : simulink/Sources/Repeating Sequence Interpolated  OutValues=|  TimeValues=|  LookUpMeth=Interpolation-Use End Values  tsamp=-1  OutMin=[]  OutMax=[]  OutDataTypeStr=double  OutputDataTypeScalingMode=double  OutDataType=fixdt(0,8)  OutScaling=2^-10
      OutValues=|
      | [  -11.1291
      |   -11.1588
      |   -11.2754
      |   -11.3348
      |   -11.3640
      |   -11.3349
      |   -11.2761
      |   -11.3644
      |   -11.4820
      |   -11.6877
      |   -11.9824
      |   -12.3084
      |   -12.4564
      |   -12.7586
      |   -12.9110
      |   -13.1851
      |   -13.3978
      |   -13.7036
      |   -13.6713
      |   -14.1054
      |   -13.8875
      |   -13.7327
      |   -13.6400
      |   -13.6400
      |   -13.7636
      |   -13.8879
      |   -14.1072
      |   -14.3577
      |   -14.5135
      |   -14.6391
      |   -14.6391
      |   -14.3243
      |   -14.2618
      |   -14.0769
      |   -13.3678
      |   -13.1847
      |   -13.1874
      |   -12.8845
      |   -12.1952
      |   -12.1968
      |   -11.7508
      |   -11.6376
      |   -11.1100
      |   -10.7030
      |   -10.1258
      |    -9.5609
      |    -9.5616
      |    -9.1089
      |    -8.8274
      |    -8.6038
      |    -8.0754
      |    -7.9926
      |    -7.0311
      |    -6.4872
      |    -6.3536
      |    -6.0586
      |    -5.7638
      |    -5.5768
      |    -5.2566
      |    -5.2045
      |    -4.5670
      |    -3.8272
      |    -3.7990
      |    -3.8776
      |    -3.7724
      |    -3.8777
      |    -4.3791
      |    -4.7245
      |    -4.5643
      |    -4.8546
      |    -5.4121
      |    -5.8135
      |    -6.1916
      |    -6.5106
      |    -6.7813
      |    -7.1642
      |    -7.2707
      |    -7.4860
      |    -7.6777
      |    -7.7616
      |    -8.1494
      |    -8.2612
      |    -9.1811
      |    -9.5460
      |   -10.2024
      |   -10.1740
      |   -10.7173
      |   -11.6519
      |   -11.9196
      |   -13.5221
      |   -14.0461
      |   -14.9577
      |   -15.4698
      |   -15.7285
      |   -16.0525
      |   -16.2152
      |   -16.2152
      |   -16.52].'
      TimeValues=|
      | [         0
      |     0.1500
      |     0.3000
      |     0.4500
      |     1.0000
      |     1.1500
      |     1.3000
      |     1.4500
      |     2.0000
      |     2.1500
      |     2.3000
      |     2.4500
      |     3.0000
      |     3.1500
      |     3.3000
      |     3.4500
      |     4.0000
      |     4.1500
      |     4.3000
      |     4.4500
      |     5.0000
      |     5.1500
      |     5.3000
      |     5.4500
      |     6.0000
      |     6.1500
      |     6.3000
      |     6.4500
      |     7.0000
      |     7.1500
      |     7.3000
      |     7.4500
      |     8.0000
      |     8.1500
      |     8.3000
      |     8.4500
      |     9.0000
      |     9.1500
      |     9.3000
      |     9.4500
      |    10.0000
      |    10.1500
      |    10.3000
      |    10.4500
      |    11.0000
      |    11.1500
      |    11.3000
      |    11.4500
      |    12.0000
      |    12.1500
      |    12.3000
      |    12.4500
      |    13.0000
      |    13.1500
      |    13.3000
      |    13.4500
      |    14.0000
      |    14.1500
      |    14.3000
      |    14.4500
      |    15.0000
      |    15.1500
      |    15.3000
      |    15.4500
      |    16.0000
      |    16.1500
      |    16.3000
      |    16.4500
      |    17.0000
      |    17.1500
      |    17.3000
      |    17.4500
      |    18.0000
      |    18.1500
      |    18.3000
      |    18.4500
      |    19.0000
      |    19.1500
      |    19.3000
      |    19.4500
      |    20.0000
      |    20.1500
      |    20.3000
      |    20.4500
      |    21.0000
      |    21.1500
      |    21.3000
      |    21.4500
      |    22.0000
      |    22.1500
      |    22.3000
      |    22.4500
      |    23.0000
      |    23.1500
      |    23.3000
      |    23.4500
      |    23.900  
      |    24.000].'
  Tout : Outport  InitialOutput=0
  wires:
  Heater Switch1/1 -> Sum2/1  "Toutdoors"
  Temp_aux/1 -> Heater Switch1/1
  Summer/1 -> Heater Switch1/2
  Heater Switch2/1 -> Sum2/2  "Toutdoors"
  Temp_aux1/1 -> Heater Switch2/1
  Winter/1 -> Heater Switch2/2
  Sum2/1 -> Tout/1
